simulink model "net_modeling"  (R2021a)
settings: Solver=VariableStepAuto  StartTime=0.0  StopTime=10.0  RelTol=1e-3
undefined symbols (not defined in the file): A
settings Model: Creator=zzy  LastModifiedBy=zzy

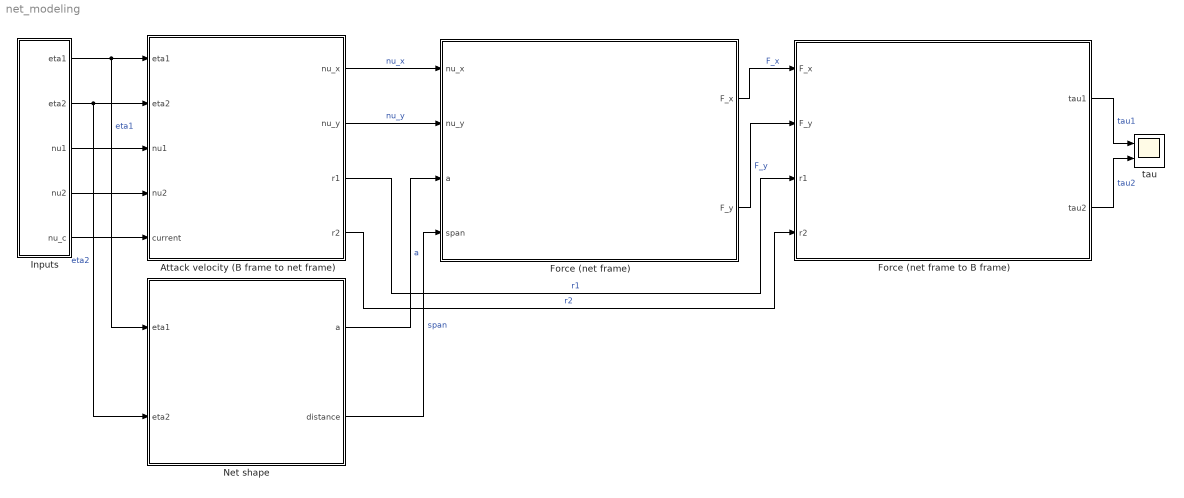
== system net_modeling ==
  Attack velocity (B frame to net frame) : MATLAB Function  TreatAsAtomicUnit=on
  Force (net frame to B frame) : MATLAB Function  TreatAsAtomicUnit=on
  Force (net frame) : MATLAB Function  TreatAsAtomicUnit=on
  Inputs : Subsystem
  Net shape : Subsystem
      mask Display: image('$imagefile'); % Use "Edit Image" on toolstrip to change.
  tau : Scope  NumInputPorts=2
  wires:
  Attack velocity (B frame to net frame)/4(r2) -> Force (net frame to B frame)/4(r2)  "r2"
  Attack velocity (B frame to net frame)/3(r1) -> Force (net frame to B frame)/3(r1)  "r1"
  Force (net frame)/1(F_x) -> Force (net frame to B frame)/1(F_x)  "F_x"
  Attack velocity (B frame to net frame)/2(nu_y) -> Force (net frame)/2(nu_y)  "nu_y"
  Force (net frame)/2(F_y) -> Force (net frame to B frame)/2(F_y)  "F_y"
  Attack velocity (B frame to net frame)/1(nu_x) -> Force (net frame)/1(nu_x)  "nu_x"
  Force (net frame to B frame)/1(tau1) -> tau/1  "tau1"
  Force (net frame to B frame)/2(tau2) -> tau/2  "tau2"
  Inputs/1(eta1) -> Attack velocity (B frame to net frame)/1(eta1), Net shape/1(eta1)  "eta1"
  Inputs/5(nu_c) -> Attack velocity (B frame to net frame)/5(current)
  Inputs/4(nu2) -> Attack velocity (B frame to net frame)/4(nu2)
  Inputs/3(nu1) -> Attack velocity (B frame to net frame)/3(nu1)
  Inputs/2(eta2) -> Attack velocity (B frame to net frame)/2(eta2), Net shape/2(eta2)  "eta2"
  Net shape/1(a) -> Force (net frame)/3(a)  "a"
  Net shape/2(distance) -> Force (net frame)/4(span)  "span"

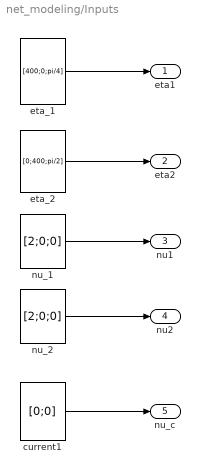
== system net_modeling/Inputs ==
  current1 : Constant  Value=[0;0]  VectorParams1D=off
  eta_1 : Constant  Value=[400;0;pi/4]  VectorParams1D=off
  eta_2 : Constant  Value=[0;400;pi/2]  VectorParams1D=off
  nu_1 : Constant  Value=[2;0;0]  VectorParams1D=off
  nu_2 : Constant  Value=[2;0;0]  VectorParams1D=off
  eta1 : Outport
  eta2 : Outport  Port=2
  nu1 : Outport  Port=3
  nu2 : Outport  Port=4
  nu_c : Outport  Port=5
  wires:
  nu_1/1 -> nu1/1
  eta_2/1 -> eta2/1
  nu_2/1 -> nu2/1
  current1/1 -> nu_c/1
  eta_1/1 -> eta1/1

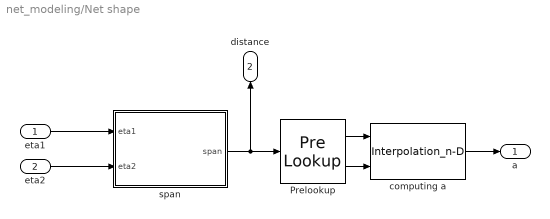
== system net_modeling/Net shape ==
  eta1 : Inport
  eta2 : Inport  Port=2
  Prelookup : PreLookup  BreakpointsData=[200:10:750]  ExtrapMethod=Linear
  computing a : Interpolation_n-D  NumberOfTableDimensions=1  Table=A  InternalRulePriority=Speed
      settings: InputPortMap=u0,u1
  span : MATLAB Function  TreatAsAtomicUnit=on
  a : Outport
  distance : Outport  Port=2
  wires:
  eta1/1 -> span/1(eta1)
  Prelookup/1 -> computing a/1
  eta2/1 -> span/2(eta2)
  Prelookup/2 -> computing a/2
  computing a/1 -> a/1
  span/1(span) -> Prelookup/1, distance/1

== matlab function net_modeling/Attack velocity (B frame to net frame) ==
  data: eta1 input; nu_x output; nu_y output; eta2 input; nu1 input; nu2 input; r1 output; r2 output; current input
function [nu_x, nu_y, r1, r2] = Attack_velocity(eta1, eta2, nu1, nu2, current)
n = 20;
nu_x = zeros(n-1,1);
nu_y = zeros(n-1,1);
psi1 = eta1(3);
psi2 = eta2(3);
eta_d = eta2 - eta1;
alpha = atan2(eta_d(2),eta_d(1)) - pi/2; % net orientation

if abs((psi1+psi2)/2-alpha) > pi/2
    alpha = -alpha;
end

r1 = alpha - psi1;
r2 = alpha - psi2;

B = [cos(r1) sin(r1) 0 0; 
        -sin(r1) cos(r1) 0 0;
        0 0 cos(r2) sin(r2);
        0 0 -sin(r2) cos(r2)];
      
R1 = [cos(psi1), sin(psi1);
          -sin(psi1), cos(psi1)];       
R2 = [cos(psi2), sin(psi2);
          -sin(psi2),cos(psi2)];

nu_c1 = R1*current;
nu_c2 = R2*current;

nu = B * [nu1(1)-nu_c1(1);  % nu1_x
                 nu1(2)-nu_c1(2);  % nu1_y
                 nu2(1)-nu_c2(1);  % nu2_x
                 nu2(2)-nu_c2(2)]; % nu2_y
 for i = 1 : n-1
    delta = [nu(3)-nu(1);
                   nu(4)-nu(2)]/(n-1);
    nu_x(i) = nu(3) - (i-0.5) * delta(1);
    nu_y(i) = nu(4) - (i-0.5) * delta(2);
 end
 
end

== matlab function net_modeling/Net shape/span ==
  data: eta1 input; span output; eta2 input
function span = dis(eta1, eta2)
pos1 = eta1(1:2);
pos2 = eta2(1:2);
span = norm(pos1-pos2);

== matlab function net_modeling/Force (net frame) ==
  data: nu_x input; F_x output; nu_y input; a input; span input; F_y output
function [F_x, F_y]= Force(nu_x, nu_y, a, span)
n = 20;
rho= 1027;
dep = 3; 
d_w = 2.5e-3; 
L = 50e-3; 
Sn = d_w*(2*L+0.5*d_w)/L^2;
D = 0.5;
draft = 0.2*D;
Cd= 1;
F_x = 0;
F_y = 0;

delta_x = span/(n-1);
X = span/2-0.5*delta_x : -delta_x: -span/2+0.5*delta_x;
 for i = 1 : (n-1)
     k = atan(sinh(X(i)/a));
     beta = atan2(nu_y(i), nu_x(i));
     theta = k + beta;
     kappa = theta - beta;
     V = nu_x(i)/cos(beta);
     C_D = 0.04+(-0.04+0.33*Sn+6.54*Sn^2-4.88*Sn^3)*cos(theta);
     C_L = (-0.05*Sn+2.3*Sn^2-1.76*Sn^3)*sin(2*theta);
     F_d1 = 0.5 * C_D * rho * V * abs(V) * dep * delta_x / cos(k); % net drag
     F_l1 = 0.5 * C_L * rho * V * abs(V) * dep * delta_x / cos(k); % net lift
     F_d = 0.5 * Cd * rho * V * cos(theta) * abs(V * cos(theta)) * 0.2 * draft * delta_x / cos(k); % buyo drag
     
     F_x = F_x + F_d1*cos(beta) + F_l1 * sin(beta) + F_d * cos(kappa); 
     F_y = F_y +  F_d1*sin(beta) - F_l1 *cos(beta) - F_d * sin(kappa);
 end

== matlab function net_modeling/Force (net frame to B frame) ==
  data: F_x input; tau1 output; F_y input; r1 input; r2 input; tau2 output
function [tau1,tau2] = Transformation(F_x, F_y, r1, r2)
B = [cos(r1) sin(r1) 0 0; 
        -sin(r1) cos(r1) 0 0;
        0 0 cos(r2) sin(r2);
        0 0 -sin(r2) cos(r2)];
drag = -[F_x/2;F_y/2;F_x/2;F_y/2];
tau = inv(B) * drag;
tau1 = tau(1:2);
tau2 = tau(3:4);
